simulink model "ComfortMdFlow"  (R2018b)
settings: Solver=FixedStepDiscrete  StartTime=0.0  StopTime=10.0  FixedStep=0.01  RelTol=1e-3
settings Model: Creator=sn2xws  LastModifiedBy=sn55gm
settings Model: ModifiedHistory=|
  | 2024.4.29 First Release
  | 2024.6.19 V1.1.0模式流程V1.6
  | 2024.8.8 V3.0.0单元测试问题修复
  | 2025.11.03 V4.0.0 修改流程，腿托只发送目标位置
settings DataIOCC: SaveFormat=StructureWithTime
settings OptimizationCC: DefaultParameterBehavior=Inlined  EnhancedBackFolding=on  PassReuseOutputArgsAs=Individual arguments  ZeroExternalMemoryAtStartup=off  ZeroInternalMemoryAtStartup=off  OptimizeBlockOrder=speed  DifferentSizesBufferReuse=on  OptimizationCustomize=off
settings DebuggingCC: ParameterTunabilityLossMsg=error
settings SFSimCC: MATLABDynamicMemAlloc=off
settings RTWCC: SystemTargetFile=autosar.tlc  GenCodeOnly=on  TemplateMakefile=ert_default_tmf  Description=AUTOSAR  GenerateReport=on  IncludeHyperlinkInReport=on  LaunchReport=on  GenerateTraceInfo=on  GenerateTraceReport=on  GenerateTraceReportSl=on  GenerateTraceReportSf=on  GenerateTraceReportEml=on
settings CodeAppCC: ForceParamTrailComments=on  IgnoreCustomStorageClasses=off  OperatorAnnotations=on  SimulinkDataObjDesc=on  SFDataObjDesc=on  InsertBlockDesc=on
settings STFCustomTargetCC: TargetLangStandard=C99 (ISO)  MultiwordLength=256  ParMdlRefBuildCompliant=on  CompOptLevelCompliant=on  IncludeMdlTerminateFcn=off  CombineOutputUpdateFcns=on  SuppressErrorStatus=on  ERTCustomFileBanners=on  SupportNonFinite=off  SupportComplex=off  SupportContinuousTime=off  SupportNonInlinedSFcns=off  RemoveResetFunc=on  MATLABClassNameForMDSCustomization=Simulink.SoftwareTarget.ERTCustomization  AutosarCompliant=on  UseToolchainInfoCompliant=on  LookupTableObjectStructAxisOrder=2,1,3,4,...  LUTObjectStructOrderEvenSpacing=Size,Table,Breakpoints  SystemTargetFile=autosar.tlc
settings ERTTargetCC: TargetLangStandard=C99 (ISO)  ConcurrentExecutionCompliant=off  IncludeMdlTerminateFcn=off  SuppressErrorStatus=on  SupportNonFinite=off  SupportComplex=off  ModelStepFunctionPrototypeControlCompliant=off  CPPClassGenCompliant=off  AutosarCompliant=on  LookupTableObjectStructAxisOrder=2,1,3,4,...  LUTObjectStructOrderEvenSpacing=Size,Table,Breakpoints  InlinedParameterPlacement=NonHierarchical  ERTCustomFileTemplate=example_file_process.tlc  ERTFilePackagingFormat=Compact

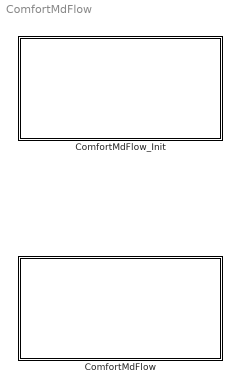
== system ComfortMdFlow ==
  ComfortMdFlow : Subsystem
  ComfortMdFlow_Init : Subsystem

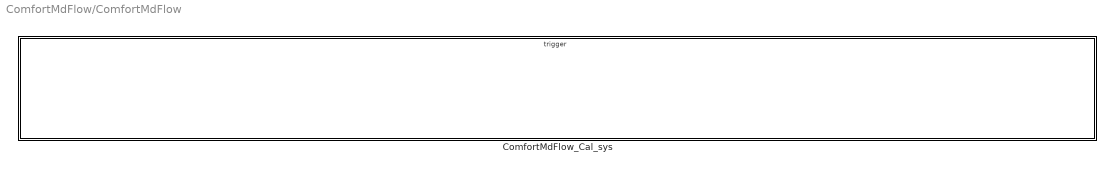
== system ComfortMdFlow/ComfortMdFlow ==
  ComfortMdFlow_Cal_sys : Subsystem

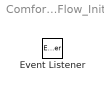
== system ComfortMdFlow/ComfortMdFlow_Init ==
  Event Listener : EventListener  EventName=reset

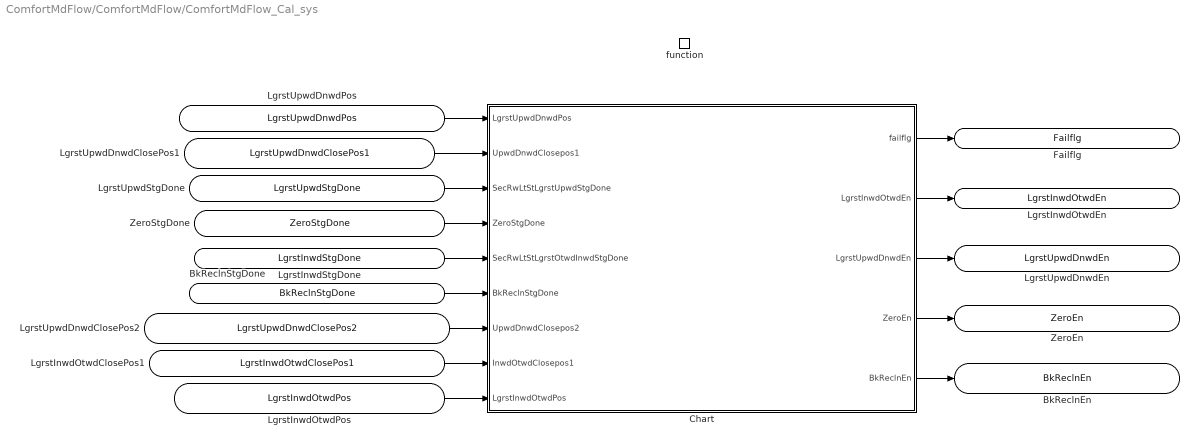
== system ComfortMdFlow/ComfortMdFlow/ComfortMdFlow_Cal_sys ==
  function : TriggerPort  TriggerType=function-call  IsSimulinkFunction=on  FunctionName=ComfortMdFlow_Cal  VariantControl=(inherit)
  Chart : Stateflow chart  TreatAsAtomicUnit=on
  LgrstUpwdDnwdPos : ArgIn  OutDataTypeStr=uint16  ArgumentName=LgrstUpwdDnwdPos
  LgrstUpwdStgDone : ArgIn  Port=2  OutDataTypeStr=boolean  ArgumentName=LgrstUpwdStgDone
  ZeroStgDone : ArgIn  Port=3  OutDataTypeStr=boolean  ArgumentName=ZeroStgDone
  LgrstInwdStgDone : ArgIn  Port=4  OutDataTypeStr=boolean  ArgumentName=LgrstInwdStgDone
  BkReclnStgDone : ArgIn  Port=5  OutDataTypeStr=boolean  ArgumentName=BkReclnStgDone
  LgrstUpwdDnwdClosePos1 : ArgIn  Port=6  OutDataTypeStr=uint16  ArgumentName=LgrstUpwdDnwdClosePos1
  LgrstUpwdDnwdClosePos2 : ArgIn  Port=7  OutDataTypeStr=uint16  ArgumentName=LgrstUpwdDnwdClosePos2
  LgrstInwdOtwdClosePos1 : ArgIn  Port=8  OutDataTypeStr=uint16  ArgumentName=LgrstInwdOtwdClosePos1
  LgrstInwdOtwdPos : ArgIn  Port=9  OutDataTypeStr=uint16  ArgumentName=LgrstInwdOtwdPos
  Failflg : ArgOut  OutDataTypeStr=boolean  ArgumentName=Failflg
  LgrstInwdOtwdEn : ArgOut  Port=2  OutDataTypeStr=boolean  ArgumentName=LgrstInwdOtwdEn
  LgrstUpwdDnwdEn : ArgOut  Port=3  OutDataTypeStr=boolean  ArgumentName=LgrstUpwdDnwdEn
  ZeroEn : ArgOut  Port=4  OutDataTypeStr=boolean  ArgumentName=ZeroEn
  BkReclnEn : ArgOut  Port=5  OutDataTypeStr=boolean  ArgumentName=BkReclnEn
  wires:
  LgrstUpwdDnwdPos/1 -> Chart/1(LgrstUpwdDnwdPos)
  LgrstUpwdDnwdClosePos1/1 -> Chart/2(UpwdDnwdClosepos1)
  LgrstUpwdStgDone/1 -> Chart/3(SecRwLtStLgrstUpwdStgDone)
  LgrstInwdStgDone/1 -> Chart/5(SecRwLtStLgrstOtwdInwdStgDone)
  ZeroStgDone/1 -> Chart/4(ZeroStgDone)
  BkReclnStgDone/1 -> Chart/6(BkReclnStgDone)
  Chart/1(failflg) -> Failflg/1
  Chart/2(LgrstInwdOtwdEn) -> LgrstInwdOtwdEn/1
  Chart/3(LgrstUpwdDnwdEn) -> LgrstUpwdDnwdEn/1
  Chart/4(ZeroEn) -> ZeroEn/1
  Chart/5(BkReclnEn) -> BkReclnEn/1
  LgrstUpwdDnwdClosePos2/1 -> Chart/7(UpwdDnwdClosepos2)
  LgrstInwdOtwdClosePos1/1 -> Chart/8(InwdOtwdClosepos1)
  LgrstInwdOtwdPos/1 -> Chart/9(LgrstInwdOtwdPos)

== stateflow chart ComfortMdFlow/ComfortMdFlow_Cal_sys/Chart ==
  (default) -> (junction 220) : {
      | failflg =0;
      | LgrstInwdOtwdEn=0;
      | LgrstUpwdDnwdEn=0;
      | BkReclnEn = 0;
      | ZeroEn = 0;
      | }
  (junction 220) -> (junction 222) [order 1] : [SecRwLtStLgrstOtwdInwdStgDone]
  (junction 220) -> (junction 226) [order 2] : {
      | LgrstInwdOtwdEn=1;
      | }
  (junction 222) -> (junction 224)
  (junction 224) -> (junction 226)
  (junction 226) -> (junction 105)
  (junction 105) -> (junction 107) [order 1] : [SecRwLtStLgrstUpwdStgDone]
  (junction 105) -> (junction 82) [order 2] : {
      | LgrstUpwdDnwdEn=1;
      | }
  (junction 107) -> (junction 109)
  (junction 109) -> (junction 82)
  (junction 82) -> (junction 166)
  (junction 166) -> (junction 202) [order 1] : [BkReclnStgDone]
  (junction 166) -> (junction 206) [order 2] : {
      | BkReclnEn=1;
      | }
  (junction 202) -> (junction 204)
  (junction 204) -> (junction 206)
  (junction 206) -> (junction 209)
  (junction 209) -> (junction 211) [order 1] : [ZeroStgDone]
  (junction 209) -> (junction 215) [order 2] : {
      | ZeroEn = 1;
      | }
  (junction 211) -> (junction 213)
  (junction 213) -> (junction 215)
  (junction 215) -> (junction 218)
  data: LgrstUpwdDnwdPos input uint16; UpwdDnwdClosepos1 input uint16; SecRwLtStLgrstUpwdStgDone input boolean; ZeroStgDone input boolean; SecRwLtStLgrstOtwdInwdStgDone input boolean; failflg output boolean; LgrstInwdOtwdEn output boolean; LgrstUpwdDnwdEn output boolean; ZeroEn output boolean; BkReclnStgDone input boolean; BkReclnEn output boolean; UpwdDnwdClosepos2 input uint16; InwdOtwdClosepos1 input uint16; LgrstInwdOtwdPos input uint16
